simulink subsystem "patient_model"  (R2019b)
settings: Solver=VariableStepAuto  StartTime=0.0  StopTime=10.0  RelTol=1e-3
undefined symbols (not defined in the file): C_v_CO2_0, C_v_O2_0, Q_0
libraries: simulink x1
(part 2 of 2)

== system patient_model/cvs_bkst/ODEs/Vessel pressure control (ap) ==
  Qin : Inport
  Qout : Inport  Port=2
  c_ : Inport  Port=3
  Add4 : Sum  Inputs=+-
  Product4 : Product  Inputs=*/
  dP_ : Outport
  wires:
  Add4/1 -> Product4/1
  Qin/1 -> Add4/1
  c_/1 -> Product4/2
  Product4/1 -> dP_/1  "dP_"
  Qout/1 -> Add4/2

== system patient_model/cvs_bkst/ODEs/Vessel pressure control (as) ==
  Qin : Inport
  Qout : Inport  Port=2
  c_ : Inport  Port=3
  Add4 : Sum  Inputs=+-
  Product4 : Product  Inputs=*/
  dP_ : Outport
  wires:
  Qout/1 -> Add4/2
  Product4/1 -> dP_/1  "dP_"
  c_/1 -> Product4/2
  Qin/1 -> Add4/1
  Add4/1 -> Product4/1

== system patient_model/cvs_bkst/ODEs/Vessel pressure control (vs) ==
  Qin : Inport
  Qout : Inport  Port=2
  c_ : Inport  Port=3
  Add4 : Sum  Inputs=+-
  Product4 : Product  Inputs=*/
  dP_ : Outport
  wires:
  Qout/1 -> Add4/2
  Product4/1 -> dP_/1  "dP_"
  c_/1 -> Product4/2
  Qin/1 -> Add4/1
  Add4/1 -> Product4/1

== system patient_model/rs_tehrani/ODEs/Ambient air pressure (-H2O) ==
  QT12 : Inport
  PA;H2O [mmHg] : Constant  Value=47
  Subtract : Sum  Inputs=+-
  Output : Outport
  wires:
  Subtract/1 -> Output/1  "Pamb*"
  PA;H2O [mmHg]/1 -> Subtract/2
  QT12/1 -> Subtract/1  "Pamb"

== system patient_model/rs_tehrani/ODEs/Insipired gas pressures ==
  Pamb* : Inport  Unit=mmHg
  Fi;O2 : Inport  Port=2  Unit=1
  Fi;CO2 : Inport  Port=3  Unit=1
  Product : Product  Inputs=**
  Product1 : Product  Inputs=**
  Pi;O2 : Outport  Unit=mmHg
  Pi;CO2 : Outport  Port=2  Unit=mmHg
  wires:
  Pamb*/1 -> Product1/1, Product/1
  Product1/1 -> Pi;CO2/1  "Pi;CO2"
  Product/1 -> Pi;O2/1  "Pi;O2"
  Fi;O2/1 -> Product/2
  Fi;CO2/1 -> Product1/2

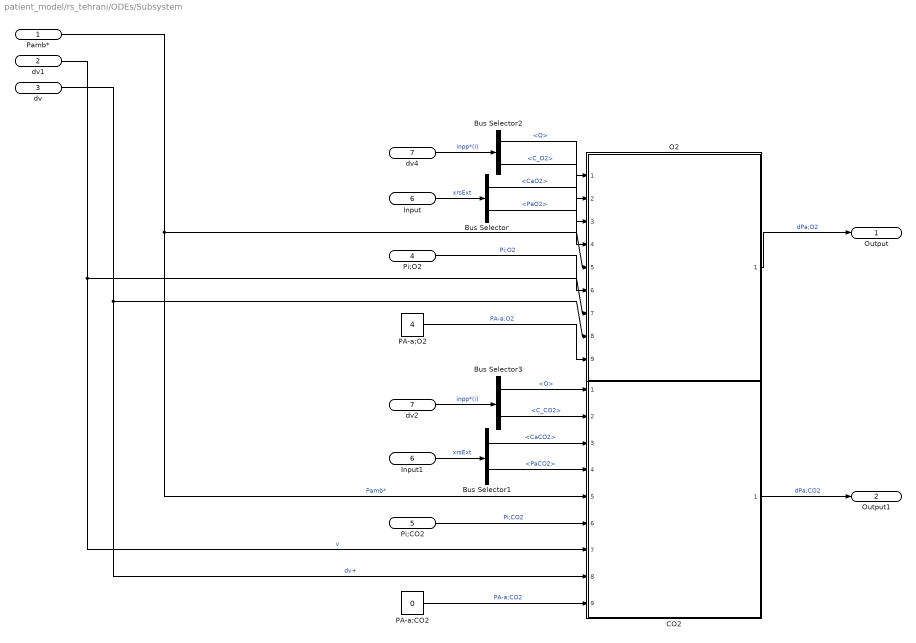
== system patient_model/rs_tehrani/ODEs/Subsystem ==
  Pamb* : Inport  Unit=mmHg
  dv1 : Inport  Port=2  Unit=L
  dv : Inport  Port=3  Unit=L/s
  Pi;O2 : Inport  Port=4  Unit=mmHg
  Pi;CO2 : Inport  Port=5  Unit=mmHg
  Input : Inport  Port=6  OutDataTypeStr=Bus: RespiratoryStateExtended
  dv4 : Inport  Port=7  OutDataTypeStr=Bus: BloodGasFlow
  Bus Selector : BusSelector  OutputSignals=CaO2,PaO2
  Bus Selector1 : BusSelector  OutputSignals=CaCO2,PaCO2
  Bus Selector2 : BusSelector  OutputSignals=Q,C_O2
  Bus Selector3 : BusSelector  OutputSignals=Q,C_CO2
  CO2 : Subsystem  ReferencedSubsystem=tehrani_alv_mass_balance_v5
  Input1 : InportShadow  Port=6  OutDataTypeStr=Bus: RespiratoryStateExtended
  O2 : Subsystem  ReferencedSubsystem=tehrani_alv_mass_balance_v5
  PA-a;CO2 : Constant  Value=0
  PA-a;O2 : Constant  Value=4
  dv2 : InportShadow  Port=7  OutDataTypeStr=Bus: BloodGasFlow
  Output : Outport  Unit=mmHg/s
  Output1 : Outport  Port=2  Unit=mmHg/s
  wires:
  PA-a;O2/1 -> O2/9  "PA-a;O2"
  Pamb*/1 -> O2/5, CO2/5  "Pamb*"
  dv/1 -> O2/8, CO2/8  "dv+"
  Pi;O2/1 -> O2/6  "Pi;O2"
  dv1/1 -> O2/7, CO2/7  "v"
  Bus Selector/2 -> O2/4  "<PaO2>"
  CO2/1 -> Output1/1  "dPa;CO2"
  PA-a;CO2/1 -> CO2/9  "PA-a;CO2"
  Bus Selector/1 -> O2/3  "<CaO2>"
  O2/1 -> Output/1  "dPa;O2"
  Bus Selector1/2 -> CO2/4  "<PaCO2>"
  Input/1 -> Bus Selector/1  "xrsExt"
  Bus Selector3/2 -> CO2/2  "<C_CO2>"
  Bus Selector3/1 -> CO2/1  "<Q>"
  dv2/1 -> Bus Selector3/1  "inpp*(i)"
  Input1/1 -> Bus Selector1/1  "xrsExt"
  dv4/1 -> Bus Selector2/1  "inpp*(i)"
  Bus Selector1/1 -> CO2/3  "<CaCO2>"
  Pi;CO2/1 -> CO2/6  "Pi;CO2"
  Bus Selector2/2 -> O2/2  "<C_O2>"
  Bus Selector2/1 -> O2/1  "<Q>"

== system patient_model/Lung volume model/Inspiratory lung volume derivative (fourier approximation)/Half-wave rectifier/summand (k=2) ==
  In1 : Inport
  In2 : Inport  Port=2
  Add1 : Sum  Inputs=+-
  Constant2 : Constant
  Product : Product
  Product3 : Product  Inputs=*/
  Square : Math  Operator=square  SignedPower=off  SaturateOnIntegerOverflow=on
  Trigonometric Function1 : Trigonometry  Operator=cos
  Out1 : Outport
  wires:
  Constant2/1 -> Add1/2
  Product3/1 -> Out1/1
  Product/1 -> Trigonometric Function1/1
  In2/1 -> Square/1, Product/2  "n"
  In1/1 -> Product/1  "omega*t"
  Square/1 -> Add1/1
  Trigonometric Function1/1 -> Product3/1
  Add1/1 -> Product3/2

== system patient_model/Lung volume model/Inspiratory lung volume derivative (fourier approximation)/Half-wave rectifier/summand (k=4) ==
  In1 : Inport
  In2 : Inport  Port=2
  Add1 : Sum  Inputs=+-
  Constant2 : Constant
  Product : Product
  Product3 : Product  Inputs=*/
  Square : Math  Operator=square  SignedPower=off  SaturateOnIntegerOverflow=on
  Trigonometric Function1 : Trigonometry  Operator=cos
  Out1 : Outport
  wires:
  Add1/1 -> Product3/2
  Trigonometric Function1/1 -> Product3/1
  Square/1 -> Add1/1
  In1/1 -> Product/1  "omega*t"
  In2/1 -> Product/2, Square/1  "n"
  Product/1 -> Trigonometric Function1/1
  Product3/1 -> Out1/1
  Constant2/1 -> Add1/2

== system patient_model/Lung volume model/Inspiratory lung volume derivative (fourier approximation)/Half-wave rectifier/summand (k=6) ==
  In1 : Inport
  In2 : Inport  Port=2
  Add1 : Sum  Inputs=+-
  Constant2 : Constant
  Product : Product
  Product3 : Product  Inputs=*/
  Square : Math  Operator=square  SignedPower=off  SaturateOnIntegerOverflow=on
  Trigonometric Function1 : Trigonometry  Operator=cos
  Out1 : Outport
  wires:
  Constant2/1 -> Add1/2
  Product3/1 -> Out1/1
  Product/1 -> Trigonometric Function1/1
  In2/1 -> Square/1, Product/2  "n"
  In1/1 -> Product/1  "omega*t"
  Square/1 -> Add1/1
  Trigonometric Function1/1 -> Product3/1
  Add1/1 -> Product3/2

== system patient_model/cvs_bkst/ODEs/Heart contractility control/Enabled Subsystem ==
  In1 : Inport
  Enable : EnablePort
  Out1 : Outport
  wires:
  In1/1 -> Out1/1

== system patient_model/cvs_bkst/ODEs/Heart contractility control/Enabled Subsystem1 ==
  In1 : Inport
  Enable : EnablePort
  Out1 : Outport
  wires:
  In1/1 -> Out1/1

== system patient_model/cvs_bkst/ODEs/Heart contractility control/Subsystem ==
  <SL> : Inport
  <sigmaL> : Inport  Port=2
  <H> : Inport  Port=3
  contrL : Inport  Port=4
  Add : Sum  Inputs=-+-
  Demux : Demux  Outputs=3
  Derivative : Derivative
  Divide : Product  Inputs=*/
  Gain : Gain  Commented=through  Gain=60
  Product : Product
  Product1 : Product
  Out1 : Outport
  wires:
  <H>/1 -> Product1/2
  Divide/1 -> Out1/1
  <sigmaL>/1 -> Derivative/1
  Derivative/1 -> Gain/1
  Demux/3 -> Divide/2
  Demux/2 -> Product1/1
  <SL>/1 -> Product/2
  Demux/1 -> Product/1
  Add/1 -> Divide/1
  Product/1 -> Add/1
  Product1/1 -> Add/2
  Gain/1 -> Add/3
  contrL/1 -> Demux/1

== system patient_model/cvs_bkst/ODEs/Heart contractility control/Subsystem1 ==
  <SL> : Inport
  <sigmaL> : Inport  Port=2
  <H> : Inport  Port=3
  contrL : Inport  Port=4
  Add : Sum  Inputs=-+-
  Demux : Demux  Outputs=3
  Derivative : Derivative
  Divide : Product  Inputs=*/
  Gain : Gain  Commented=through  Gain=60
  Product : Product
  Product1 : Product
  Out1 : Outport
  wires:
  contrL/1 -> Demux/1
  Gain/1 -> Add/3
  Product1/1 -> Add/2
  Product/1 -> Add/1
  Add/1 -> Divide/1
  Demux/1 -> Product/1
  <SL>/1 -> Product/2
  Demux/2 -> Product1/1
  Demux/3 -> Divide/2
  Derivative/1 -> Gain/1
  <sigmaL>/1 -> Derivative/1
  Divide/1 -> Out1/1
  <H>/1 -> Product1/2

== system patient_model/cvs_bkst/ODEs/Systemic vascular resistance control/Subsystem ==
  dRs [0] : Inport
  dRs [v] : Inport  Port=2
  dRs [a] : Inport  Port=3
  Constant : Constant  Value=0
  Constant1 : Constant
  Constant2 : Constant  Value=2
  Equal : RelationalOperator  Operator===  OutDataTypeStr=boolean  RndMeth=Simplest
  Equal1 : RelationalOperator  Operator===  OutDataTypeStr=boolean  RndMeth=Simplest
  Equal2 : RelationalOperator  Operator===  OutDataTypeStr=boolean  RndMeth=Simplest
  Merge : Merge  Inputs=3
  Rs calculation mode : Constant  Value=2
  Subsystem1 : Subsystem
  Subsystem2 : Subsystem
  Subsystem3 : Subsystem
  dRs : Outport  Unit=mmHg/L
  wires:
  dRs [v]/1 -> Subsystem2/1(in)  "dRs;mode1"
  Subsystem1/1(out) -> Merge/3
  Equal2/1 -> Subsystem1/Enable
  Merge/1 -> dRs/1  "dRs"
  Rs calculation mode/1 -> Equal/2, Equal1/2, Equal2/2
  dRs [0]/1 -> Subsystem3/1(in)  "dRs;mode0"
  Equal/1 -> Subsystem3/Enable
  Constant/1 -> Equal/1
  Subsystem2/1(out) -> Merge/2
  Equal1/1 -> Subsystem2/Enable
  dRs [a]/1 -> Subsystem1/1(in)  "dRs;mode2"
  Constant1/1 -> Equal1/1
  Constant2/1 -> Equal2/1
  Subsystem3/1(out) -> Merge/1

== system patient_model/cvs_bkst/ODEs/Systemic vascular resistance control/Subsystem/Subsystem1 ==
  in : Inport
  Enable : EnablePort
  out : Outport
  wires:
  in/1 -> out/1

== system patient_model/cvs_bkst/ODEs/Systemic vascular resistance control/Subsystem/Subsystem2 ==
  in : Inport
  Enable : EnablePort
  out : Outport
  wires:
  in/1 -> out/1

== system patient_model/cvs_bkst/ODEs/Systemic vascular resistance control/Subsystem/Subsystem3 ==
  in : Inport
  Enable : EnablePort
  out : Outport
  wires:
  in/1 -> out/1
